simulink library "DigiConLib"  (Simulink 9.0)
settings: Solver=VariableStepAuto  StartTime=0.0  StopTime=10.0  RelTol=1e-3
libraries: realtime_pacer_lib x1
settings Model: Creator=alexandersoussan  LastModifiedBy=Danny

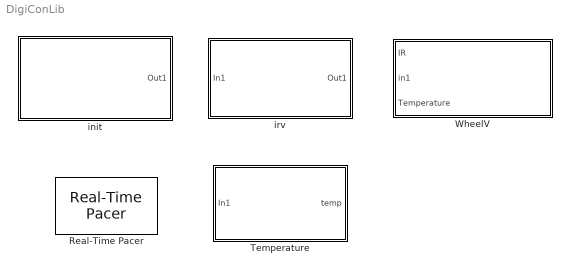
== system DigiConLib ==
  Real-Time Pacer : realtime_pacer_lib/Real-Time Pacer  simTimePerRealTime=0.5
  Temperature : Subsystem
  WheelV : Subsystem
  init : Subsystem
  irv : Subsystem

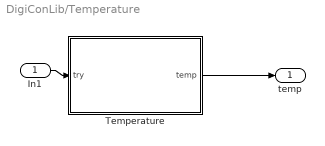
== system DigiConLib/Temperature ==
  In1 : Inport
  Temperature : Stateflow chart  TreatAsAtomicUnit=on
  temp : Outport
  wires:
  Temperature/1(temp) -> temp/1
  In1/1 -> Temperature/1(try)

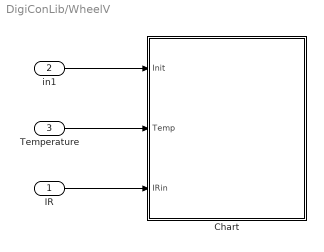
== system DigiConLib/WheelV ==
  IR : Inport
  in1 : Inport  Port=2
  Temperature : Inport  Port=3
  Chart : Stateflow chart  TreatAsAtomicUnit=on
  wires:
  IR/1 -> Chart/3(IRin)
  Temperature/1 -> Chart/2(Temp)
  in1/1 -> Chart/1(Init)

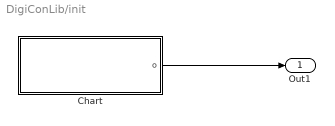
== system DigiConLib/init ==
  Chart : Stateflow chart  TreatAsAtomicUnit=on
  Out1 : Outport
  wires:
  Chart/1(o) -> Out1/1

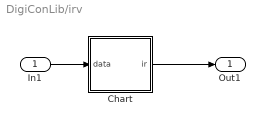
== system DigiConLib/irv ==
  In1 : Inport
  Chart : Stateflow chart  TreatAsAtomicUnit=on
  Out1 : Outport
  wires:
  Chart/1(ir) -> Out1/1
  In1/1 -> Chart/1(data)

== stateflow chart irv/Chart ==
  state RANGE
    en,du:
    ir=irv
  (default) -> RANGE
  data: rState function_output double; ir output double; data input int8
  function rState = irv:
    | function rState = irv
    | rState = [0,0,0,0,0,0];
    | persistent objB
    | coder.extrinsic('evalin')
    | if isempty(objB)
    |     objB = evalin('base','objWs')
    | end
    | coder.extrinsic('RangeStateRoomba')
    | rState = RangeStateRoomba(objB);

== stateflow chart Temperature/Temperature ==
  state temp
    en,du:
    temp=Temper;
  (default) -> temp
  data: y function_output double; try input double; temp output double
  function y= Temper:
    | function y= Temper
    | persistent so
    | y=1;
    | coder.extrinsic('evalin');
    | coder.extrinsic('get');
    | 
    | so = evalin('base','objWs');
    | 
    | temp=0;  
    | coder.extrinsic('TemperatureRoomba');
    | temp=TemperatureRoomba(so);
    | 
    | y=temp;

== stateflow chart init/Chart ==
  state A1
    en:
    tcpInit;
    o = 1;
  (default) -> A1
  data: o output double
  function tcpInit:
    | function tcpInit
    | persistent obj
    | coder.extrinsic('RoombaWiFiInit');
    | coder.extrinsic('assignin');
    | obj=RoombaWiFiInit('10.0.0.1','full');
    | assignin('base','objWs',obj);

== stateflow chart WheelV/Chart ==
  state Begin1
    state off
      en,du:
      WheelV(0,0);
    state on
      state GoBack
        entry:
        WheelV(-0.2,-0.2);
      state GoForward
        entry,du:
        WheelV(0.05,0.05);
      state Rightturn3
        entry,du:
        WheelV(-0.2,0.2);
      state leftturn3
        entry,du:
        WheelV(0.2,-0.2);
      state Leftturn3
        entry,du:
        WheelV(0.3,-0.2);
      state turn_right2
        entry,du:
        WheelV(-0.2,0.3);
      state Leftturn2
        entry,du:
        WheelV(0.2,-0.1);
      state SharpRight
        entry,du:
        WheelV(-0.1,0.2);
      (default) -> GoBack
      GoBack -> GoForward : after(1,sec)
      GoForward -> Rightturn3 [order 3] : [IRin(3)>0]
      Rightturn3 -> GoForward : [IRin(3)<1]
      GoForward -> leftturn3 [order 4] : [IRin(4)>0]
      leftturn3 -> GoForward : [IRin(4)<1]
      GoForward -> Leftturn3 [order 5] : [(IRin(5)>0)&&(IRin(6)>0)]
      Leftturn3 -> GoForward : [(IRin(5)<1)&&(IRin(6)<1)]
      GoForward -> Leftturn2 [order 6] : [(IRin(5)>0)|(IRin(6)>0)]
      Leftturn2 -> GoForward : [(IRin(5))&&(IRin(6)<1)]
      GoForward -> SharpRight [order 1] : [(IRin(1)>0)|(IRin(2)>0)]
      SharpRight -> GoForward : [(IRin(1)<1)&&(IRin(2)<1)]
      GoForward -> turn_right2 [order 2] : [(IRin(1)>0)&&(IRin(2)>0)]
      turn_right2 -> GoForward : [(IRin(1)<1)&&(IRin(2)<1)]
    (default) -> off
    off -> on : [Temp<80]
    on -> off : [Temp>=80]
  (default) -> Begin1
  data: u1 function_input double; u2 function_input double; Init input double; Temp input double; IRin input double
  function WheelV(u1,u2):
    | function WheelV(u1,u2)
    | persistent so
    | coder.extrinsic('evalin');
    | coder.extrinsic('get');
    | so = evalin('base','objWs');
    | coder.extrinsic('SetWheelVelRoomba');
    | SetWheelVelRoomba(so,u1,u2);
